simulink model "problem3_dummy"  (R2015b)
settings: Solver=VariableStepAuto  StartTime=0.0  StopTime=20  RelTol=1e-3
settings Model: Creator=kjartan  LastModifiedBy=kjartan

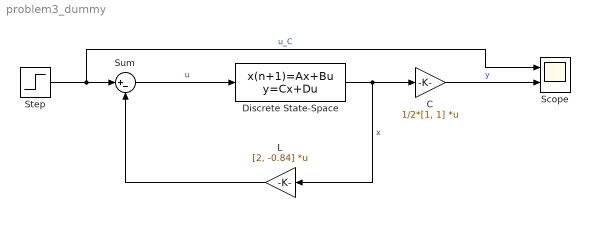
== system problem3_dummy ==
  C : Gain  Gain=1/2*[1, 1]  Multiplication=Matrix(K*u) (u vector)
  Discrete State-Space : DiscreteStateSpace  A=[2, -1; 1, 0]  B=[1;0]  C=eye(2)  D=[0;0]
  L : Gain  Gain=[2, -0.84]  Multiplication=Matrix(K*u) (u vector)
  Scope : Scope  NumInputPorts=2
  Step : Step  SampleTime=0
  Sum : Sum  Inputs=|+-
  wires:
  Step/1 -> Scope/1, Sum/1  "u_C"
  Discrete State-Space/1 -> L/1, C/1  "x"
  L/1 -> Sum/2
  Sum/1 -> Discrete State-Space/1  "u"
  C/1 -> Scope/2  "y"
